simulink model "ADPSEStaF1LEMK"  (R2018b)
settings: Solver=ode1  StartTime=0.0  StopTime=10  FixedStep=1/1000  RelTol=1e-3  AbsTol=1e-3  EnableMultiTasking=on
PostLoadFcn:
  | f_Simulink_figureplace
InitFcn:
  | ADPSEStaF1LEMK_PreSim
values from neighbouring files (symbols this model uses):
  beta = 0.003    [ADPSEStaF1LEMK_PreSim.m]
  d1 = s*[0;1]    [ADPSEStaF1LEMK_PreSim.m]
  d2 = s*[0.8660;-0.5]    [ADPSEStaF1LEMK_PreSim.m]
  d3 = s*[-0.8660;-0.5]    [ADPSEStaF1LEMK_PreSim.m]
  dbar = 0.00001    (= 1e-05)    [ADPSEStaF1LEMK_PreSim.m]
  etaa1 = 1.2    [ADPSEStaF1LEMK_PreSim.m]
  etaa2 = 0.01    [ADPSEStaF1LEMK_PreSim.m]
  etac1 = 0.001    [ADPSEStaF1LEMK_PreSim.m]
  etac2 = 0.25    [ADPSEStaF1LEMK_PreSim.m]
  Gamma0 = 250*eye(L)    [ADPSEStaF1LEMK_PreSim.m]
  MovePoints = 1    [ADPSEStaF1LEMK_PreSim.m]
  NormBas = 0    [ADPSEStaF1LEMK_PreSim.m]
  NormDyn = 0    [ADPSEStaF1LEMK_PreSim.m]
  Q = [1 0 ; 0 1]    [ADPSEStaF1LEMK_PreSim.m]
  R = 1    [ADPSEStaF1LEMK_PreSim.m]
  s = 0.7    [ADPSEStaF1LEMK_PreSim.m]
  v = 0.05    [ADPSEStaF1LEMK_PreSim.m]
  v2 = 1    [ADPSEStaF1LEMK_PreSim.m]
  WaH0 = 0.7*WcH0    [ADPSEStaF1LEMK_PreSim.m]
  WcH0 = 0.4*[1 1 1]'    [ADPSEStaF1LEMK_PreSim.m]
  x0 = [-1;1]    [ADPSEStaF1LEMK_PreSim.m]
settings Model: Creator=rkamalapurkar  LastModifiedBy=rushik
settings SolverCC: AutoScaleAbsTol=off
settings DataIOCC: SaveFormat=StructureWithTime  SaveOutput=off  DSMLogging=off  SaveTime=off  SignalLoggingName=ADPCLStaF
settings OptimizationCC: ExpressionDepthLimit=2147483647  LifeSpan=inf
settings DebuggingCC: UnderspecifiedInitializationDetection=Classic  MergeDetectMultiDrivingBlocksExec=none  SolverPrmCheckMsg=warning  FcnCallInpInsideContextMsg=warning  StateNameClashWarn=warning  SFUnexpectedBacktrackingDiag=warning  SFNoUnconditionalDefaultTransitionDiag=warning  SFExecutionAtInitializationDiag=none
settings HardwareCC: ProdBitPerPointer=32  ProdBitPerSizeT=32  ProdBitPerPtrDiffT=32  ProdLargestAtomicFloat=None  ProdIntDivRoundTo=Undefined  ProdEndianess=Unspecified  ProdWordSize=32  ProdHWDeviceType=32-bit Generic
settings ModelReferenceCC: PropagateSignalLabelsOutOfModel=off
settings SFSimCC: SimUseLocalCustomCode=off
settings RTWCC: RTWUseLocalCustomCode=off
settings CodeAppCC: StateflowObjectComments=on
settings GRTTargetCC: TargetLangStandard=C89/C90 (ANSI)  GeneratePreprocessorConditionals=Disable all  CombineOutputUpdateFcns=off  GRTInterface=on
settings ConfigComp: CovMetricSettings=dw  CovHtmlReporting=on  CovSaveCumulativeToWorkspaceVar=on  CovSaveSingleToWorkspaceVar=on  CovExternalEMLEnable=off  CovSFcnEnable=off

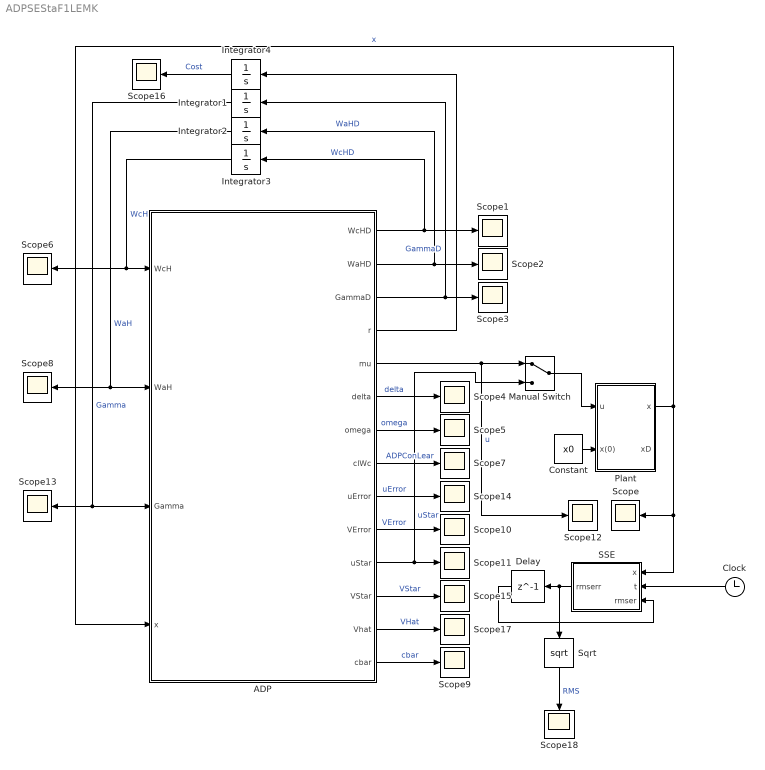
== system ADPSEStaF1LEMK ==
  ADP : MATLAB Function  TreatAsAtomicUnit=on
  Clock : Clock
  Constant : Constant  Value=x0
  Delay : Delay  DelayLength=1  InitialCondition=0
  Integrator1 : Integrator  InitialCondition=Gamma0
  Integrator2 : Integrator  InitialCondition=WaH0
  Integrator3 : Integrator  InitialCondition=WcH0
  Integrator4 : Integrator
  Manual Switch : ManualSwitch
  Plant : Subsystem
  SSE : MATLAB Function  TreatAsAtomicUnit=on
  Scope{,1..18} (19 alike) : Scope
  Sqrt : Sqrt  SaturateOnIntegerOverflow=on
  wires:
  ADP/3(GammaD) -> Integrator1/1, Scope3/1  "GammaD"
  ADP/1(WcHD) -> Integrator3/1, Scope1/1  "WcHD"
  Integrator3/1 -> ADP/1(WcH), Scope6/1  "WcH"
  ADP/2(WaHD) -> Integrator2/1, Scope2/1  "WaHD"
  Integrator2/1 -> ADP/2(WaH), Scope8/1  "WaH"
  ADP/6(delta) -> Scope4/1  "delta"
  ADP/7(omega) -> Scope5/1  "omega"
  Integrator1/1 -> ADP/3(Gamma), Scope13/1  "Gamma"
  ADP/5(mu) -> Manual Switch/1, Scope12/1  "u"
  ADP/8(clWc) -> Scope7/1  "ADPConLear"
  Plant/1(x) -> ADP/4(x), SSE/1(x), Scope/1  "x"
  Constant/1 -> Plant/2(x(0))
  ADP/9(uError) -> Scope14/1  "uError"
  ADP/14(cbar) -> Scope9/1  "cbar"
  ADP/10(VError) -> Scope10/1  "VError"
  ADP/11(uStar) -> Manual Switch/2, Scope11/1  "uStar"
  ADP/12(VStar) -> Scope15/1  "VStar"
  ADP/13(Vhat) -> Scope17/1  "VHat"
  Manual Switch/1 -> Plant/1(u)
  Integrator4/1 -> Scope16/1  "Cost"
  ADP/4(r) -> Integrator4/1
  Clock/1 -> SSE/2(t)
  SSE/1(rmserr) -> Sqrt/1, Delay/1
  Delay/1 -> SSE/3(rmser)
  Sqrt/1 -> Scope18/1  "RMS"

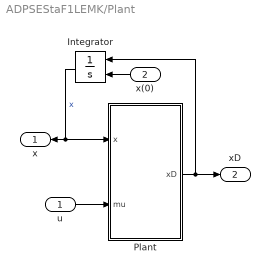
== system ADPSEStaF1LEMK/Plant ==
  u : Inport
  x(0) : Inport  Port=2
  Integrator : Integrator  InitialConditionSource=external  InitialCondition=[1;1;0.0;0.0]
  Plant : MATLAB Function  TreatAsAtomicUnit=on
  x : Outport
  xD : Outport  Port=2
  wires:
  Plant/1(xD) -> Integrator/1, xD/1
  Integrator/1 -> Plant/1(x), x/1  "x"
  u/1 -> Plant/2(mu)
  x(0)/1 -> Integrator/2

== matlab function ADPSEStaF1LEMK/Plant/Plant ==
  data: xD output; x input; mu input
function xD = dynamics(x,mu)
%#codegen
F=[-x(1)+x(2) ;-0.5*x(1)-0.5*x(2)*(1-(cos(2*x(1))+2)^2)];
G=[0; (cos(2*x(1))+2)];
xD = F+G*mu;

== matlab function ADPSEStaF1LEMK/ADP ==
  settings: updateMethod=DISCRETE
  data: WcH input; WaH input; Gamma input; x input; R parameter; Q parameter; etaa1 parameter; etaa2 parameter; v2 parameter; s parameter; dbar parameter; d1 parameter; d2 parameter; d3 parameter; etac1 parameter; etac2 parameter; v parameter; WcHD output; WaHD output; GammaD output; r output; mu output; delta output; omega output; clWc output; uError output; VError output; uStar output; beta parameter; MovePoints parameter; VStar output; Vhat output; cbar output; NormBas parameter; NormDyn parameter; x0 parameter
function [WcHD,WaHD,GammaD,r,mu,delta,omega,clWc,uError,VError,uStar,VStar,Vhat,cbar]=...
    control(WcH,WaH,Gamma,x,R,Q,etaa1,etaa2,v2,s,dbar,d1,d2,d3,...
    etac1,etac2,v,beta,MovePoints,NormBas,NormDyn,x0)
%#codegen

if NormDyn == 1
    a = norm(x0);
else
    a = 1;
end
n=2;
thetaS=[-1 1 -0.5 -0.5]'; % True values of SysID Parameters
y = x/a;
G = [0 ; (cos(2*a*y(1))+2)]./a;
Y = [a*y(1) a*y(2) 0 0;0 0 a*y(1) a*y(2)*(1-(cos(2*a*y(1))+2)^2)]./a;
[sig,sig_p] = ADPSEStaF1LEMK_Basis(y,d1,d2,d3,v2,dbar,NormBas);
mu=-0.5*(R\G')*sig_p'*WaH;

theta = thetaS;%*(model==1) + thetaH*(model~=1);
%% Concurrent Learning
nm=(y'*y+dbar)/(1+v2*(y'*y));
if MovePoints == 0
    temp=linspace(-3*s*nm,3*s*nm,5);
    [temp1, temp2] = ndgrid(temp,temp);
    XC=[temp1(:) temp2(:)]'; % matrix with columns as selected points
    M = length(temp)^n; %Number of points
else
    M=1;
    XC=unifrnd(-3*s*nm,3*s*nm,n,M);
% XC1=sin(2*pi*t) + sin(exp(1)*t) + cos(5*t)^5;
% XC2=sin(5*pi*t) + sin(exp(8)*t) + cos(2*t)^5;
% XC3=sin(4*pi*t) + sin(exp(1.4)*t) + cos(1*t)^5;
% XC4=sin(5*pi*t) + sin(exp(1.3)*t) + cos(0.5*t)^5;
% XC5=sin(3*pi*t) + sin(exp(1.1)*t) + cos(10*t)^5;
% XC6=sin(2*pi*t) + sin(exp(1.8)*t) + cos(11*t)^5;
% XC=[XC1;XC2];
end
clWc=zeros(size(WcH));
clWa=zeros(size(WaH));
CLmatrix=zeros(size(WcH,1),size(WcH,1));
CLGamma=zeros(size(Gamma));
parfor i=1:M
    xi=y+XC(:,i);
    [~,sig_pi] = ADPSEStaF1LEMK_Basis(xi,d1,d2,d3,v2,dbar,NormBas);   
    Gi = [0 ; (cos(2*xi(1))+2)]./a;
    Yi = [xi(1) xi(2) 0 0;0 0 xi(1) xi(2)*(1-(cos(2*xi(1))+2)^2)]./a;
    mui=-0.5*(R\Gi')*sig_pi'*WaH;
    omegai = sig_pi*(Yi*theta+Gi*mui);
    rhoi=(1+v*(omegai'*omegai));
    ri = xi'*Q*xi*a^2 + mui'*R*mui;
    deltai = WcH'*omegai + ri;
    clWc=clWc+Gamma*omegai*deltai/rhoi;
    Gsigmai = sig_pi*Gi*(R\Gi')*sig_pi';
    clWa=clWa+Gsigmai'*WaH*omegai'*WcH/(4*rhoi);
    CLmatrix=CLmatrix+omegai*omegai'/(M*rhoi);
    CLGamma=CLGamma+Gamma*(omegai*omegai'/rhoi^2)*Gamma;
end
clWc=-etac2*clWc/M;
clWa=etac2*clWa/M;
CLGamma=CLGamma/M;
cbar=min(svd(CLmatrix));
%% ADP
omega = sig_p*(Y*theta+G*mu);
Gsigma = sig_p*G*(R\G')*sig_p';
r = y'*Q*y*a^2 + mu'*R*mu;
delta = WcH'*omega + r;
rho = (1+v*(omega'*omega));
WcHD = (-etac1*Gamma*omega*delta/rho+clWc);
GammaD = (beta*Gamma-Gamma*(omega*omega'/rho^2)*Gamma-CLGamma);
WaHD = etaa1*(WcH-WaH)...
    -(etaa2*WaH-etac1*Gsigma'*WaH*omega'*WcH/(4*rho))+clWa;

uStar=-(cos(2*x(1))+2)*x(2);
uError=uStar-mu;
VStar=(1/2)*x(1)^2+x(2)^2;
Vhat = WcH'*sig;
VError=VStar-Vhat;

== matlab function ADPSEStaF1LEMK/SSE ==
  data: x input; t input; rmser input; rmserr output
function rmserr = fcn(x,t,rmser)
%#codegen

if t>90
    rmserr = rmser+(1/10000)*(norm(x))^2;
else
    rmserr = 0;
end
